simulink subsystem "F550_Dynamic_CA"  (R2024a)
settings: Solver=VariableStepAuto  StartTime=0.0  StopTime=10.0  RelTol=1e-3
values from neighbouring files (symbols this model uses):
  Jxx = 0.0211    [F550_data.m]
  Jyy = 0.0219    [F550_data.m]
  Jzz = 0.0366    [F550_data.m]
  Mass = 2.06    [F550_data.m]
libraries: matrix_library x1
settings Model: Creator=UASG  LastModifiedBy=UASG

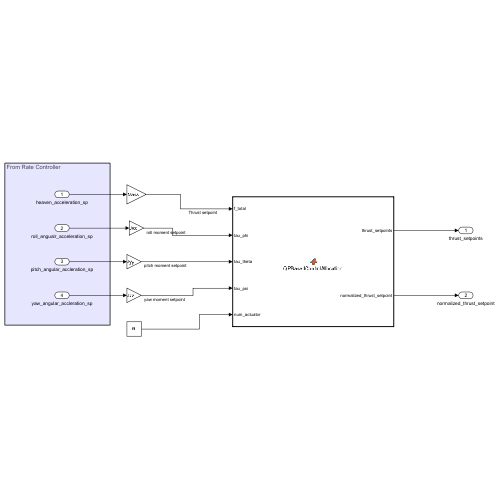
[thumbnail: Simulink's stored preview of the top-level diagram]
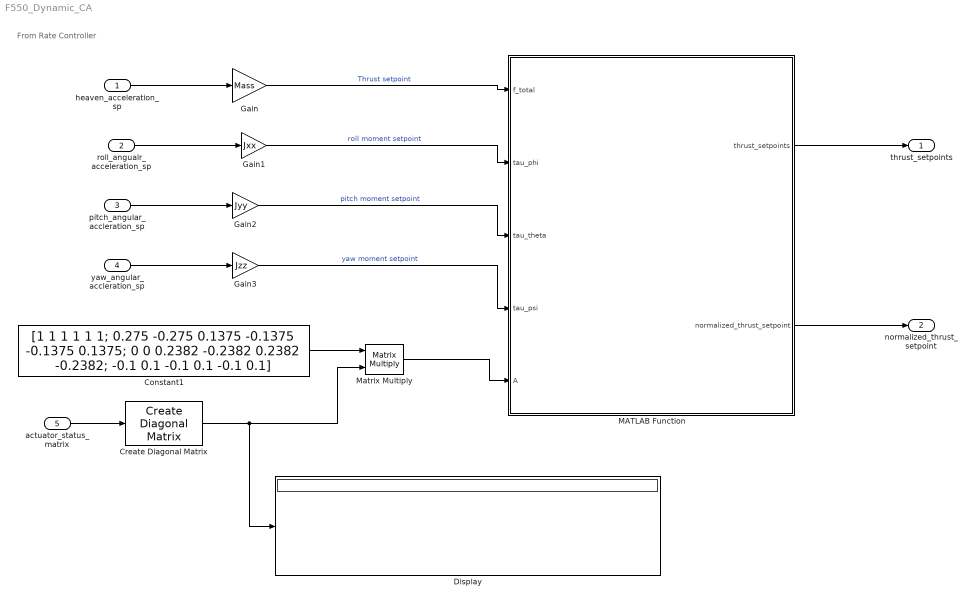
== system F550_Dynamic_CA ==
  note: From Rate Controller
  heaven_acceleration_sp : Inport
  roll_angualr_acceleration_sp : Inport  Port=2
  pitch_angular_accleration_sp : Inport  Port=3
  yaw_angular_accleration_sp : Inport  Port=4
  actuator_status_matrix : Inport  Port=5
  Constant1 : Constant  Value=[1 1 1 1 1 1; 0.275 -0.275 0.1375 -0.1375 -0.1375 0.1375; 0 0 0.2382 -0.2382 0.2382 -0.2382; -0.1 0.1 -0.1 0.1 -0.1 0.1]
  Create Diagonal Matrix : matrix_library/Create Diagonal Matrix
      settings: LibrarySourceBlock=|
      | simulink/Matrix
      | Operations/Create Diagonal
      | Matrix
  Display : Display
  Gain : Gain  Gain=Mass
  Gain1 : Gain  Gain=Jxx
  Gain2 : Gain  Gain=Jyy
  Gain3 : Gain  Gain=Jzz
  MATLAB Function : MATLAB Function  TreatAsAtomicUnit=on
  Matrix Multiply : Product  Multiplication=Matrix(*)
  thrust_setpoints : Outport
  normalized_thrust_setpoint : Outport  Port=2
  wires:
  heaven_acceleration_sp/1 -> Gain/1
  Gain/1 -> MATLAB Function/1(f_total)  "Thrust setpoint"
  roll_angualr_acceleration_sp/1 -> Gain1/1
  Gain1/1 -> MATLAB Function/2(tau_phi)  "roll moment setpoint"
  pitch_angular_accleration_sp/1 -> Gain2/1
  Gain2/1 -> MATLAB Function/3(tau_theta)  "pitch moment setpoint"
  yaw_angular_accleration_sp/1 -> Gain3/1
  Gain3/1 -> MATLAB Function/4(tau_psi)  "yaw moment setpoint"
  MATLAB Function/1(thrust_setpoints) -> thrust_setpoints/1
  MATLAB Function/2(normalized_thrust_setpoint) -> normalized_thrust_setpoint/1
  actuator_status_matrix/1 -> Create Diagonal Matrix/1
  Constant1/1 -> Matrix Multiply/1
  Create Diagonal Matrix/1 -> Matrix Multiply/2, Display/1
  Matrix Multiply/1 -> MATLAB Function/5(A)

== matlab function F550_Dynamic_CA/MATLAB Function ==
  data: f_total input; thrust_setpoints output; tau_phi input; tau_theta input; tau_psi input; A input; normalized_thrust_setpoint output
function [thrust_setpoints, normalized_thrust_setpoint] = QPBasedControlAllocation(f_total, tau_phi, tau_theta, tau_psi, A)
persistent prev_thrust_setpoint;

if(isempty(prev_thrust_setpoint))
    prev_thrust_setpoint = zeros(1,6);
end

% f_total: 추력 명령 [N], tau_phi, tau_theta, tau_psi: 롤 피치 요 토크 명령 [N.m]
% thrust_setpoints: 각 모터별 추력 명령[N] normalized_thrust_setpoint: 모터 최대 출력으로
% 정규화한 값
% A : Control Effectiviness MAtrix
num_actuator = 6;
u_des = [f_total; tau_phi; tau_theta; tau_psi];

% 각 추진기의 추력 제한 정의 (예시 값)
f_min = 0;           % 최소 추력 (뉴턴)
f_max = 5;           % 최대 추력 (뉴턴)

% 목적 함수의 이차 및 선형 계수 정의
% 목적: f' * f (추력의 제곱합 최소화)
H = 2 * eye(num_actuator);      % MATLAB의 quadprog은 (1/2)x'Hx + f'x를 최소화
f_obj = zeros(num_actuator,1);  % 선형 항 없음

% 등식 제약 조건: A * f = u_des
Aeq = A;
beq = u_des;

% 변수의 하한 및 상한
lb = f_min * ones(num_actuator,1);
ub = f_max * ones(num_actuator,1);

% 이차 프로그래밍 문제 해결
options = optimoptions('quadprog', 'Display','none', 'Algorithm', 'active-set');  % 출력 숨기기
[thrust_setpoints, ~, ~, ~] = quadprog(H, f_obj, [], [], Aeq, beq, lb, ub, prev_thrust_setpoint, options);
normalized_thrust_setpoint = thrust_setpoints ./ f_max;
prev_thrust_setpoint = thrust_setpoints;
